simulink subsystem "subsystem_directDynamics_rigid"  (R2022a)
settings: Solver=VariableStepAuto  StartTime=0.0  StopTime=10.0  RelTol=1e-3
settings Model: Creator=Philipp  LastModifiedBy=Philipp
settings DebuggingCC: UnconnectedInputMsg=warning  UnconnectedOutputMsg=warning  UnconnectedLineMsg=warning
settings RTWCC: DLArmComputeVersion=19.05

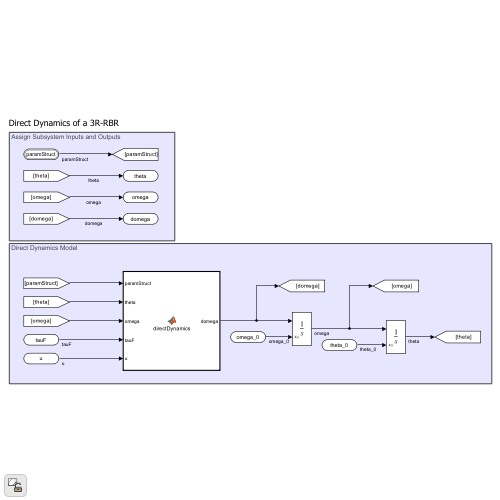
[thumbnail: Simulink's stored preview of the top-level diagram]
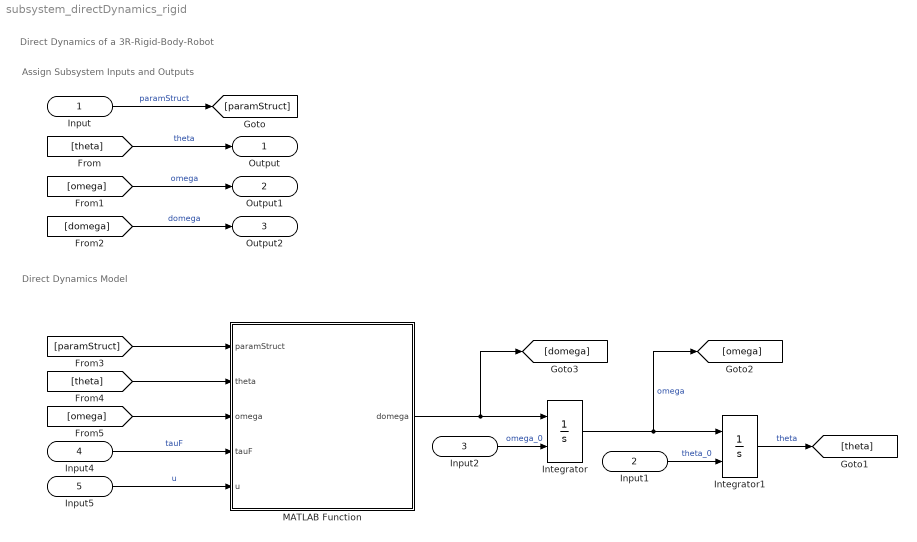
== system subsystem_directDynamics_rigid ==
  note: Direct Dynamics of a 3R-Rigid-Body-Robot
  note: Assign Subsystem Inputs and Outputs
  note: Direct Dynamics Model
  Input : Inport  OutDataTypeStr=Bus: main_bus
  Input1 : Inport  Port=2
  Input2 : Inport  Port=3
  Input4 : Inport  Port=4
  Input5 : Inport  Port=5
  Integrator : Integrator  InitialConditionSource=external
  Integrator1 : Integrator  InitialConditionSource=external
  MATLAB Function : MATLAB Function  TreatAsAtomicUnit=on
  Output : Outport
  Output1 : Outport  Port=2
  Output2 : Outport  Port=3
  wires:
  Integrator1/1 -> [theta]  "theta"
  Input1/1 -> Integrator1/2  "theta_0"
  Integrator/1 -> Integrator1/1, [omega]  "omega"
  Input2/1 -> Integrator/2  "omega_0"
  MATLAB Function/1(domega) -> [domega], Integrator/1
  Input5/1 -> MATLAB Function/5(u)  "u"
  Input4/1 -> MATLAB Function/4(tauF)  "tauF"
  [omega] -> MATLAB Function/3(omega)
  [theta] -> MATLAB Function/2(theta)
  [paramStruct] -> MATLAB Function/1(paramStruct)
  Input/1 -> [paramStruct]  "paramStruct"
  [theta] -> Output/1  "theta"
  [domega] -> Output2/1  "domega"
  [omega] -> Output1/1  "omega"

== matlab function subsystem_directDynamics_rigid/MATLAB Function ==
  data: paramStruct input; theta input; domega output; omega input; tauF input; u input
function domega = directDynamics(paramStruct, theta, omega, tauF, u)

g = paramStruct.robot.g;
r_P1P2 = paramStruct.robot.r_P1P2;
r_P2P3 = paramStruct.robot.r_P2P3;
r_P3P4 = paramStruct.robot.r_P3P4;
baseParam = paramStruct.robot.baseParam;

domega = directDynamics_rigid_fun(g, r_P1P2, r_P2P3, r_P3P4, baseParam, theta, omega, tauF, u);
